simulink model "baro_test"  (R2017b)
settings: Solver=FixedStepDiscrete  StartTime=0.0  StopTime=inf  RelTol=1e-3  EnableMultiTasking=on
libraries: beaglebonebluelib x2
settings Model: SimulationMode=external  ExtModeTrigDuration=200  Creator=pthb3  LastModifiedBy=pthb3
settings SolverCC: PositivePriorityOrder=on
settings DataIOCC: InspectSignalLogs=on
settings OptimizationCC: PassReuseOutputArgsAs=Individual arguments  MaxStackSize=64
settings DebuggingCC: ParameterTunabilityLossMsg=error
settings HardwareCC: ProdBitPerPointer=32  ProdBitPerSizeT=32  ProdBitPerPtrDiffT=32  ProdLargestAtomicInteger=Long  ProdLargestAtomicFloat=Double  ProdWordSize=32  ProdHWDeviceType=ARM Compatible->ARM Cortex
settings SFSimCC: MATLABDynamicMemAlloc=off
settings RTWCC: SystemTargetFile=ert.tlc  HardwareBoard=Raspberry Pi  TemplateMakefile=ert_default_tmf  GenerateReport=on  Toolchain=GNU GCC Raspberry Pi  IncludeHyperlinkInReport=on  LaunchReport=on  GenerateTraceInfo=on  GenerateTraceReport=on  GenerateTraceReportSl=on  GenerateTraceReportSf=on  GenerateTraceReportEml=on
settings CodeAppCC: ForceParamTrailComments=on  IgnoreCustomStorageClasses=off  OperatorAnnotations=on  SimulinkDataObjDesc=on  SFDataObjDesc=on  InsertBlockDesc=on
settings ERTTargetCC: SupportVariableSizeSignals=on

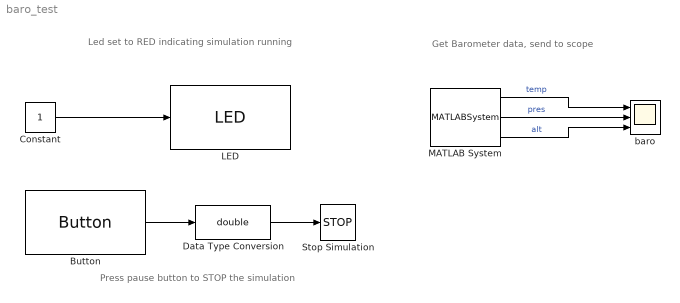
== system baro_test ==
  note: Get Barometer data, send to scope
  note: Press pause button to STOP the simulation
  note: Led set to RED indicating simulation running
  Button : beaglebonebluelib/Button  Button=Pause  SampleTime=0.01  SimulateUsing=Code generation
  Constant : Constant
  Data Type Conversion : DataTypeConversion  OutDataTypeStr=double
  LED : beaglebonebluelib/LED  LED=Red
  MATLAB System : MATLABSystem  System=beagleboneblue.bbblueBarometer  oversample=x16  filter=BMP_FILTER_16  SampleTime=0.03
      mask Type: beagleboneblue.bbblueBarometer
      mask Display:
      | color('white');
      | plot([100,100,100,100]*1,[100,100,100,100]*1);
      | plot([100,100,100,100]*0,[100,100,100,100]*0);
      | color('blue');
      | text(100, 92, ' BB BLUE ', 'horizontalAlignment', 'right');
      | color('black');
      | text(52,52,' Barometer','horizontalAlignment','center');
      | color('black');
  Stop Simulation : Stop
  baro : Scope  NumInputPorts=3
  wires:
  Constant/1 -> LED/1
  Button/1 -> Data Type Conversion/1
  MATLAB System/2 -> baro/2  "pres"
  MATLAB System/1 -> baro/1  "temp"
  MATLAB System/3 -> baro/3  "alt"
  Data Type Conversion/1 -> Stop Simulation/1
